simulink model "prueba_aislamiento_datos_corruptos"  (R2018a)
settings: Solver=VariableStepAuto  StartTime=0.0  StopTime=0.8  RelTol=1e-3
settings Model: Creator=cmparedes  LastModifiedBy=cmparedes

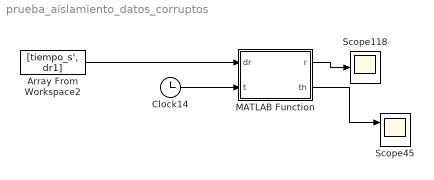
== system prueba_aislamiento_datos_corruptos ==
  Array From Workspace2 : FromWorkspace  VariableName=[tiempo_s', dr1]
  Clock14 : Clock
  MATLAB Function : MATLAB Function  TreatAsAtomicUnit=on
  Scope118 : Scope
  Scope45 : Scope  NumInputPorts=2
  wires:
  MATLAB Function/2(th) -> Scope45/1
  Clock14/1 -> MATLAB Function/2(t)
  MATLAB Function/1(r) -> Scope118/1
  Array From Workspace2/1 -> MATLAB Function/1(dr)

== matlab function prueba_aislamiento_datos_corruptos/MATLAB Function ==
  data: dr input; r output; t input; th output
function [r,th]   = fcn(dr,t)

persistent a i
if isempty(a)
    a=1;
    i=1
       
end
if t<=0.33
    th=1.5e4;
%     v=2;
else
    th=2e4;  %2e4
%     v=3;
end

r=0;
if a==2
    r=1;
end
% ra=r;

if abs(dr(1,:))>th && a==1
    r=1;
    a=a+1;
%     if v==0
%         v=1;
elseif abs(dr(1,:))>th && a==2
    r=0;
    a=1; %1
end

i=i+1
